simulink library "DCmotor_library"  (Simulink 7.4)
settings: Solver=ode45  StartTime=0.0  StopTime=10.0  RelTol=1e-3
libraries: simulink x4, rtsynclib x1
settings Model: Creator=ae  LastModifiedBy=sw

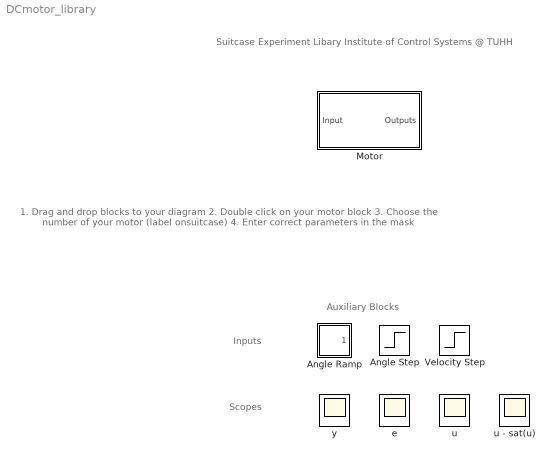
== system DCmotor_library ==
  note: Suitcase Experiment Libary
      | Institute of Control Systems @ TUHH
  note: 1. Drag and drop blocks to your diagram
      | 2. Double click on your motor block
      | 3. Choose the number of your motor (label onsuitcase)
      | 4. Enter correct parameters in the mask
  note: Auxiliary Blocks
  note: Inputs
  note: Scopes
  Angle Ramp : Subsystem  mask(Ramp){slope=1, start=1, X0=0, VectorParams1D=on, sampletime=0.01}
      mask prompts: slope "Simulink:masks:Slope_MP"; start "Simulink:masks:StartTime_MP"; X0 "Simulink:masks:InitialOutput_MP"; VectorParams1D "Simulink:masks:InterpretVectorParametersAs1D_MP"; sampletime "Sample time"
      mask help: Simulink:masks:Ramp_MD
      mask init:
      | blkName = gcb;
      | set_param([blkName '/Constant'], 'VectorParams1D',VectorParams1D);
      | set_param([blkName '/Constant1'], 'VectorParams1D',VectorParams1D);
      | set_param([blkName '/Step'], 'VectorParams1D',VectorParams1D);
      mask Display: plot([0:10],[1,1,1,1:8])
  Angle Step : Step  After=10  SampleTime=0.01
  Motor : Subsystem  InitFcn=|  StopFcn=|  mask{motoridinput=1, name_signal=Velocity, ts=10}
      InitFcn=|
      | id_tag = daq.getDevices().ID;
      | ni_obj = daq.createSession('ni');
      | ni_obj.addAnalogInputChannel(id_tag,'ai0','Voltage');
      | ni_obj.addAnalogInputChannel(id_tag,'ai1','Voltage');
      | ni_obj.addAnalogInputChannel(id_tag,'ai2','Voltage');
      | ni_obj.addAnalogInputChannel(id_tag,'ai3','Voltage');
      | ni_obj.addAnalogOutputChannel(id_tag, 'ao0', 'Voltage');
      StopFcn=|
      | ni_obj.outputSingleScan(2.5);          
      | clearvars ans id_tag jumps mvals ni_obj
      mask prompts: motoridinput "Motor Number"; name_signal "Output Variable"; ts "Sampling Time [ms]"
      mask help:
      | Select signal and corresponding units
      |
      |     Signal   |      SI     |      Motor
      | --------------------------------------------
      |    Velocity      [rad/s]         [rot/s]
      |    Angle          [rad]            [°]
      |    Current         [A]             [mA]
      |    Voltage         [V]             [V]
      mask init:
      | name_unit = 'SI'; %Motor, Raw
      | 
      | load motor.mat;
      | %global GLOB_motor
      | 
      | if ~exist('GLOB_motor')
      |     error('Please first load motor data from file motor.mat')
      | end
      | 
      | motor = GLOB_motor;
      | 
      | if strcmp(name_signal, 'Velocity')
      |     selector_signals = 1;
      | elseif strcmp(name_signal, 'Angle')
      |     selector_signals = 2;
      | elseif strcmp(name_signal, 'Current')
      |     selector_signals = 3;
      | elseif strcmp(name_signal, 'Voltage')
      |     selector_signals = 4;
      | else
      |     warning('using default: first signal')
      |     selector_signals = 1;
      | end
      | 
      | % setup DAQ object
      | % id_tag = daq.getDevices().ID;
      | % 
      | % ni_obj = daq.createSession('ni');
      | % 
      | % ni_obj.addAnalogInputChannel(id_tag,'ai0','Voltage');
      | % ni_obj.addAnalogInputChannel(id_tag,'ai1','Voltage');
      | % ni_obj.addAnalogInputChannel(id_tag,'ai2','Voltage');
      | % ni_obj.addAnalogInputChannel(id_tag,'ai3','Voltage');
      | % ni_obj.addAnalogOutputChannel(id_tag, 'ao0', 'Voltage');
      | 
      | % try
      | %    NIusb = visa('ni','USB::0x1234::125::A22-5::INSTR');
      | %    if ~strcmp(NIusb.ModelCode,'0x007D')
      | %        warning('Unknown NIDAQ model')
      | %    end
      | %    sn = NIusb.SerialNumber;
      | % catch
      | %    warning('USB device not detected automatically') 
      | %    sn = 0;
      | % end
      | % 
      | % 
      | % 
      | % if isnumeric(motoridinput)
      | %     if motoridinput == 31
      | %         if sn     
      | %             disp('Looking for known devices')
      | %             no = 1; 
      | %             while no < 31
      | %                 if strcmp(motor{no}.nidaq.serialnumber,sn)
      | %                     set_param(gcb,'motoridinput',num2str(no));
      | %                     break
      | %                 else
      | %                     no = no+1;
      | %                 end
      | %             end
      | %         else
      | %             warning('Motor could not be automatically detected - CALIBRATION for Motor 1 taken')
      | %             motorid = motor{1};
      | %         end
      | %         
      | %     elseif motoridinput == 0;
      | %   
      | %         motorid.calibration.velocity.offset = 0;
      | %         motorid.calibration.velocity.slope = 1;
      | %         motorid.calibration.angle.offset = 0;
      | %         motorid.calibration.angle.slope = 1;
      | %         motorid.calibration.current.offset = 0;
      | %         motorid.calibration.current.slope = 1;
      | %         motorid.calibration.voltage.offset = 0;
      | %         motorid.calibration.voltage.slope = 1;
      | %     elseif ((motoridinput == round(motoridinput)) & motoridinput <= 30)
      | %         if sn
      | %             if strcmp(motor{motoridinput}.nidaq.serialnumber,sn)
      | %                 motorid = motor{motoridinput};
      | %             else
      | %                 warning('Serial Number conflict: Wrong motor number given?')
      | %                 motorid = motor{motoridinput};
      | %             end
      | %         else
      | %             warning('Serial Number unknown: Calibration may be wrong')
      | %             motorid = motor{motoridinput}
      | %         end
      | %     else
      | %         error('Unknown motor ID')
      | %     end
      | % elseif isstruct(motoridinput)
      | %     disp('Using own motor ID structure')
      | % else
      | %     error('Wrong motor object - use motor number!')
      | % end
      | motorid = motor{motoridinput};
      | 
      | if strcmp(name_unit,'SI')
      |         motorid.calibration.velocity.unit = 1;
      |         motorid.calibration.angle.unit = 1;
      |         motorid.calibration.current.unit = 1;
      |         motorid.calibration.voltage.unit = 1;
      | elseif strcmp(name_unit,'Motor')
      |         motorid.calibration.velocity.unit = 2*pi;
      |         motorid.calibration.angle.unit = 180/pi;
      |         motorid.calibration.current.unit = 0.001;
      |         motorid.calibration.voltage.unit = 1;
      | elseif strcmp(name_unit,'Raw')
      |         motorid.calibration.velocity.unit = 1;
      |         motorid.calibration.angle.unit = 1;
      |         motorid.calibration.current.unit = 1;
      |         motorid.calibration.voltage.unit = 1;
      |         motorid.calibration.velocity.offset = 0;
      |         motorid.calibration.velocity.slope = 1;
      |         motorid.calibration.angle.offset = 0;
      |         motorid.calibration.angle.slope = 1;
      |         motorid.calibration.current.offset = 0;
      |         motorid.calibration.current.slope = 1;
      |         motorid.calibration.voltage.offset = 0;
      |         motorid.calibration.voltage.slope = 1;
      | else
      |     warning('Units not correct defined')
      | end
      | 
      | switch ts 
      |     % Sample Time
      |     case 1
      |         motorid.timing.sampletime = 10;
      |     case 2
      |         motorid.timing.sampletime = 20;
      |     case 3
      |         motorid.timing.sampletime = 30;
      |     case 4
      |         motorid.timing.sampletime = 50;
      |     case 5
      |         motorid.timing.sampletime = 75;
      |     case 6
      |         motorid.timing.sampletime = 100;
      |     case 7
      |         motorid.timing.sampletime = 150;
      |     otherwise
      |         error('unknown sampletime')
      | end
      | 
      | % Set the USB Port parameter
      | %tmp=daqhwinfo('nidaq');
      | 
      | %set_param([gcb,'/Analog Input'],'Device',['nidaq ' tmp.InstalledBoardIds{1} ' (USB-6008)']);
      | 
      | % Set the sampling rate
      | sr = motorid.timing.sampletime;
      | %set_param([gcb,'/motorzugriff'],'SampleRate',num2str(sr));
      | %   set_param([gcb,'/Analog Input'],'BlockSize','2');
      | 
      | 
      | % try 
      | %     % Initialize Adapter
      | %     hw = daqhwinfo;
      | %     adaptors = hw.InstalledAdaptors;
      | %     ni = daqhwinfo('nidaq');
      | %     id = ni.InstalledBoardIds;
      | %     name = ni.AdaptorName;
      | % 
      | %     % Find analog output
      | %     ao = analogoutput('nidaq',id{1});
      | %     set(ao,'SampleRate',ts);
      | %     ch = addchannel(ao,0);
      | % 
      | %     % Set corresponding motorid structure
      | %     motorid.signals.output = ao;
      | %     putsample(ao,2.5);
      | %     pause(3)
      | % catch
      | %     ao =[];
      | %     warning('No USB Board detected: Check connection')
      | % end
      mask StyleString: popup(1|2|3|4|5|6|7|8|9|10|11|12|13|14|15|16|17|18|19|20|21|22|23|24|25|26|27|28|29|30|31|32|33|34|35|36|37|38|39|40|41|42|43|44|45|46|47|48|49|50|51|52|53|54|55|56|57|58|59|60|61|62|unknown),popup(Velocity|Angle|Current|Voltage),popup(10|20|30|50|75|100|150)
      mask Display:
      | port_label('input', 1, 'Voltage')
      | port_label('output', 1, name_signal)
  Velocity Step : Step  After=47.75  SampleTime=0.01
  e : Scope
      settings: YMin=-0.5  YMax=11
  u : Scope
      settings: YMin=-0.5  YMax=11  SaveName=ScopeData2
  u - sat(u) : Scope
      settings: YMin=-0.5  YMax=11  SaveName=ScopeData3
  y : Scope
      settings: YMin=-0.5  YMax=11  SaveName=ScopeData4

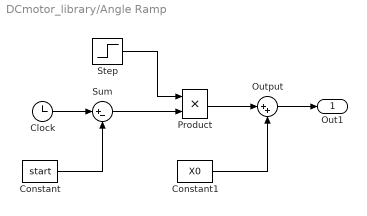
== system DCmotor_library/Angle Ramp ==
  Clock : Clock
      settings: DisableCoverage=on
  Constant : Constant  DisableCoverage=on  Value=start  OutDataTypeStr=Inherit: Inherit via back propagation
  Constant1 : Constant  DisableCoverage=on  Value=X0  OutDataTypeStr=Inherit: Inherit via back propagation
  Output : Sum  Inputs=|++  SaturateOnIntegerOverflow=on  InputSameDT=on  OutDataTypeStr=Inherit: Same as first input
  Product : Product  DisableCoverage=on  SaturateOnIntegerOverflow=on  InputSameDT=on  OutDataTypeStr=Inherit: Same as first input
  Step : Step  DisableCoverage=on  Time=start  After=slope  SampleTime=sampletime
  Sum : Sum  DisableCoverage=on  Inputs=|+-  SaturateOnIntegerOverflow=on  InputSameDT=on  OutDataTypeStr=Inherit: Same as first input
  Out1 : Outport
  wires:
  Clock/1 -> Sum/1
  Constant/1 -> Sum/2
  Sum/1 -> Product/2
  Output/1 -> Out1/1
  Constant1/1 -> Output/2
  Product/1 -> Output/1
  Step/1 -> Product/1

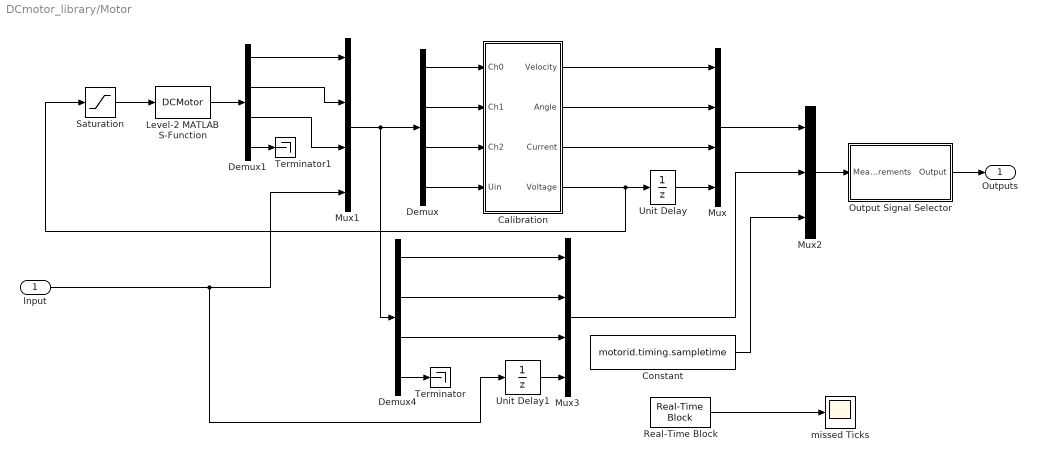
== system DCmotor_library/Motor ==
  Input : Inport
  Calibration : Subsystem
  Constant : Constant  Value=motorid.timing.sampletime
  Demux : Demux
  Demux1 : Demux
  Demux4 : Demux
  Level-2 MATLAB S-Function : M-S-Function  FunctionName=DCMotor  Parameters=ni_obj
  Mux : Mux
  Mux1 : Mux
  Mux2 : Mux  Inputs=3
  Mux3 : Mux
  Output Signal Selector : Subsystem  StopFcn=|
      | global GLOB_filename;        
      | %data.filename=GLOB_filename;
      | %data=save_data(data);
      mask Type: Output Signal Selector
      mask Description: Select the desired output.
      mask Display:
      | port_label('output',1, 'Output');
      | port_label('input' ,1 , 'Motor');
      | %port_label('input',1,['Task ' name_labproblem name_task name_subtask]);
  Real-Time Block : rtsynclib/Real-Time Block  sync_type=Fixed  sync_time=motorid.timing.sampletime*1e-3
  Saturation : Saturate  UpperLimit=5  LowerLimit=0
  Terminator : Terminator
  Terminator1 : Terminator
  Unit Delay : UnitDelay  SampleTime=-1
  Unit Delay1 : UnitDelay  SampleTime=-1
  missed Ticks : Scope
      settings: YMin=0  YMax=300
  Outputs : Outport
  wires:
  Demux4/4 -> Terminator/1
  Mux3/1 -> Mux2/2
  Unit Delay1/1 -> Mux3/4
  Demux4/3 -> Mux3/3
  Demux4/2 -> Mux3/2
  Demux4/1 -> Mux3/1
  Mux/1 -> Mux2/1
  Calibration/4(Voltage) -> Saturation/1, Unit Delay/1
  Calibration/3(Current) -> Mux/3
  Calibration/2(Angle) -> Mux/2
  Calibration/1(Velocity) -> Mux/1
  Mux1/1 -> Demux4/1, Demux/1
  Demux/1 -> Calibration/1(Ch0)
  Demux/2 -> Calibration/2(Ch1)
  Demux/3 -> Calibration/3(Ch2)
  Demux/4 -> Calibration/4(Uin)
  Demux1/1 -> Mux1/1
  Demux1/2 -> Mux1/2
  Demux1/3 -> Mux1/3
  Constant/1 -> Mux2/3
  Input/1 -> Unit Delay1/1, Mux1/4
  Unit Delay/1 -> Mux/4
  Real-Time Block/1 -> missed Ticks/1
  Mux2/1 -> Output Signal Selector/1(Measurements)
  Output Signal Selector/1(Output) -> Outputs/1
  Demux1/4 -> Terminator1/1
  Level-2 MATLAB S-Function/1 -> Demux1/1
  Saturation/1 -> Level-2 MATLAB S-Function/1

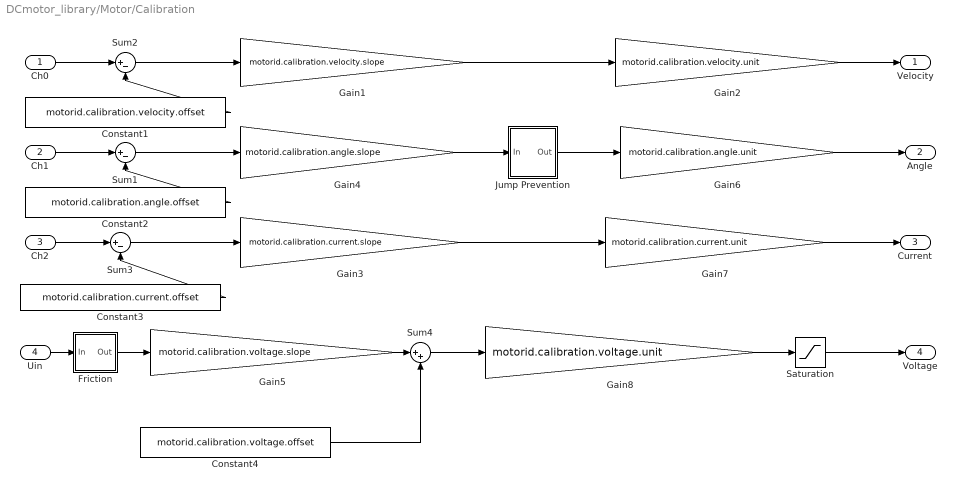
== system DCmotor_library/Motor/Calibration ==
  Ch0 : Inport
  Ch1 : Inport  Port=2
  Ch2 : Inport  Port=3
  Uin : Inport  Port=4
  Constant1 : Constant  Value=motorid.calibration.velocity.offset
  Constant2 : Constant  Value=motorid.calibration.angle.offset
  Constant3 : Constant  Value=motorid.calibration.current.offset
  Constant4 : Constant  Value=motorid.calibration.voltage.offset
  Friction : Subsystem
  Gain1 : Gain  Gain=motorid.calibration.velocity.slope
  Gain2 : Gain  Gain=motorid.calibration.velocity.unit
  Gain3 : Gain  Gain=motorid.calibration.current.slope
  Gain4 : Gain  Gain=motorid.calibration.angle.slope
  Gain5 : Gain  Gain=motorid.calibration.voltage.slope
  Gain6 : Gain  Gain=motorid.calibration.angle.unit
  Gain7 : Gain  Gain=motorid.calibration.current.unit
  Gain8 : Gain  Gain=motorid.calibration.voltage.unit
  Jump Prevention : Subsystem
  Saturation : Saturate  UpperLimit=5  LowerLimit=0
  Sum1 : Sum  Inputs=|+-
  Sum2 : Sum  Inputs=|+-
  Sum3 : Sum  Inputs=|+-
  Sum4 : Sum  Inputs=|++
  Velocity : Outport
  Angle : Outport  Port=2
  Current : Outport  Port=3
  Voltage : Outport  Port=4
  wires:
  Gain4/1 -> Jump Prevention/1(In)
  Gain8/1 -> Saturation/1
  Gain7/1 -> Current/1
  Gain6/1 -> Angle/1
  Gain2/1 -> Velocity/1
  Constant1/1 -> Sum2/2
  Constant2/1 -> Sum1/2
  Constant3/1 -> Sum3/2
  Constant4/1 -> Sum4/2
  Sum2/1 -> Gain1/1
  Ch0/1 -> Sum2/1
  Sum1/1 -> Gain4/1
  Ch1/1 -> Sum1/1
  Sum3/1 -> Gain3/1
  Ch2/1 -> Sum3/1
  Uin/1 -> Friction/1(In)
  Gain1/1 -> Gain2/1
  Gain3/1 -> Gain7/1
  Friction/1(Out) -> Gain5/1
  Sum4/1 -> Gain8/1
  Gain5/1 -> Sum4/1
  Saturation/1 -> Voltage/1
  Jump Prevention/1(Out) -> Gain6/1

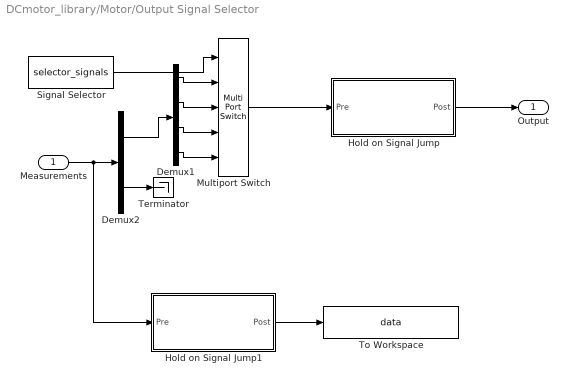
== system DCmotor_library/Motor/Output Signal Selector ==
  Measurements : Inport
  Demux1 : Demux
  Demux2 : Demux  Outputs=[4 -1]
  Hold on Signal Jump : Subsystem
  Hold on Signal Jump1 : Subsystem  AncestorBlock=DCmotor_library/Motor/Output Signal Selector/Hold on Signal Jump
  Multiport Switch : MultiPortSwitch  Inputs=4  zeroidx=off
  Signal Selector : Constant  Value=selector_signals
  Terminator : Terminator
  To Workspace : ToWorkspace  VariableName=data  SampleTime=-1  SaveFormat=Structure With Time
  Output : Outport
  wires:
  Multiport Switch/1 -> Hold on Signal Jump/1(Pre)
  Hold on Signal Jump/1(Post) -> Output/1
  Demux2/1 -> Demux1/1
  Measurements/1 -> Demux2/1, Hold on Signal Jump1/1(Pre)
  Demux1/1 -> Multiport Switch/2
  Demux1/2 -> Multiport Switch/3
  Demux1/3 -> Multiport Switch/4
  Demux1/4 -> Multiport Switch/5
  Signal Selector/1 -> Multiport Switch/1
  Demux2/2 -> Terminator/1
  Hold on Signal Jump1/1(Post) -> To Workspace/1

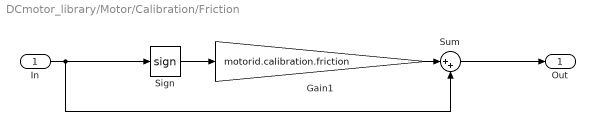
== system DCmotor_library/Motor/Calibration/Friction ==
  In : Inport
  Gain1 : Gain  DisableCoverage=on  Gain=motorid.calibration.friction  OutDataTypeStr=Inherit: Inherit via back propagation  SaturateOnIntegerOverflow=on
  Sign : Signum
  Sum : Sum  Inputs=|++  SaturateOnIntegerOverflow=on  InputSameDT=on  OutDataTypeStr=Inherit: Same as first input
  Out : Outport
  wires:
  Sum/1 -> Out/1
  Gain1/1 -> Sum/1
  In/1 -> Sign/1, Sum/2
  Sign/1 -> Gain1/1

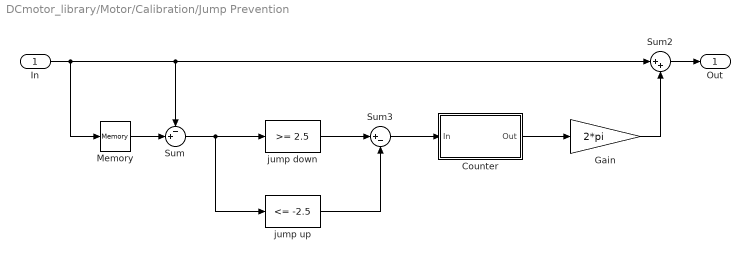
== system DCmotor_library/Motor/Calibration/Jump Prevention ==
  In : Inport
  Counter : Subsystem
  Gain : Gain  Gain=2*pi
  Memory : Memory
  Sum : Sum  Inputs=-+|
  Sum2 : Sum  Inputs=|++
  Sum3 : Sum  Inputs=|+-  OutDataTypeStr=double
  jump down : simulink/Logic and Bit Operations/Compare To Constant  relop=>=  const=2.5  LogicOutDataTypeMode=uint8  ZeroCross=off
  jump up : simulink/Logic and Bit Operations/Compare To Constant  relop=<=  const=-2.5  LogicOutDataTypeMode=uint8  ZeroCross=off
  Out : Outport
  wires:
  jump down/1 -> Sum3/1
  Sum2/1 -> Out/1
  Gain/1 -> Sum2/2
  jump up/1 -> Sum3/2
  Sum/1 -> jump up/1, jump down/1
  Memory/1 -> Sum/2
  In/1 -> Sum2/1, Sum/1, Memory/1
  Sum3/1 -> Counter/1(In)
  Counter/1(Out) -> Gain/1

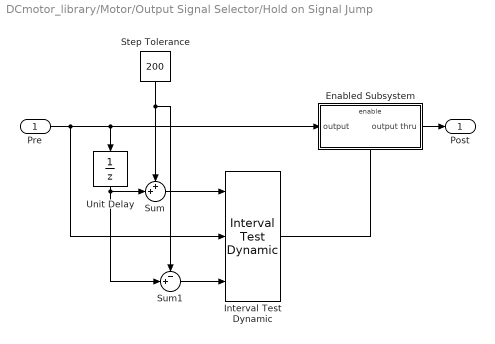
== system DCmotor_library/Motor/Output Signal Selector/Hold on Signal Jump ==
  Pre : Inport
  Enabled Subsystem : Subsystem  TreatAsAtomicUnit=on
  Interval Test Dynamic : simulink/Logic and Bit Operations/Interval Test Dynamic  IntervalClosedRight=on  IntervalClosedLeft=on  LogicOutDataTypeMode=boolean
  Step Tolerance : Constant  Value=200
  Sum : Sum  Inputs=++|
  Sum1 : Sum  Inputs=-+|
  Unit Delay : UnitDelay  SampleTime=-1
  Post : Outport
  wires:
  Enabled Subsystem/1(output thru) -> Post/1
  Pre/1 -> Enabled Subsystem/1(output), Unit Delay/1, Interval Test Dynamic/2
  Unit Delay/1 -> Sum/2, Sum1/2
  Sum/1 -> Interval Test Dynamic/1
  Sum1/1 -> Interval Test Dynamic/3
  Step Tolerance/1 -> Sum/1, Sum1/1
  Interval Test Dynamic/1 -> Enabled Subsystem/Enable

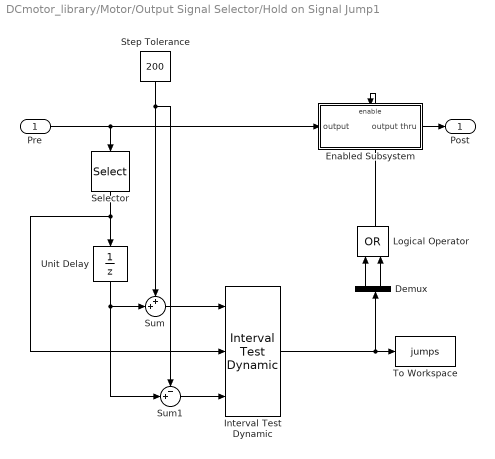
== system DCmotor_library/Motor/Output Signal Selector/Hold on Signal Jump1 ==
  Pre : Inport
  Demux : Demux  Outputs=2
  Enabled Subsystem : Subsystem  TreatAsAtomicUnit=on
  Interval Test Dynamic : simulink/Logic and Bit Operations/Interval Test Dynamic  IntervalClosedRight=on  IntervalClosedLeft=on  LogicOutDataTypeMode=boolean
  Logical Operator : Logic  Operator=OR  AllPortsSameDT=off  OutDataTypeStr=boolean
  Selector : Selector  InputPortWidth=9  IndexOptions=Index vector (dialog)  Indices=[1 2]  OutputSizes=1
  Step Tolerance : Constant  Value=200
  Sum : Sum  Inputs=++|
  Sum1 : Sum  Inputs=-+|
  To Workspace : ToWorkspace  VariableName=jumps  SampleTime=-1  SaveFormat=Structure
  Unit Delay : UnitDelay  SampleTime=-1
  Post : Outport
  wires:
  Interval Test Dynamic/1 -> To Workspace/1, Demux/1
  Step Tolerance/1 -> Sum1/1, Sum/1
  Sum1/1 -> Interval Test Dynamic/3
  Sum/1 -> Interval Test Dynamic/1
  Unit Delay/1 -> Sum1/2, Sum/2
  Pre/1 -> Enabled Subsystem/1(output), Selector/1
  Enabled Subsystem/1(output thru) -> Post/1
  Selector/1 -> Unit Delay/1, Interval Test Dynamic/2
  Demux/1 -> Logical Operator/1
  Demux/2 -> Logical Operator/2
  Logical Operator/1 -> Enabled Subsystem/Enable

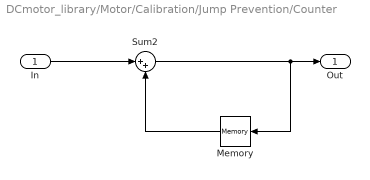
== system DCmotor_library/Motor/Calibration/Jump Prevention/Counter ==
  In : Inport
  Memory : Memory
  Sum2 : Sum  Inputs=|++
  Out : Outport
  wires:
  Sum2/1 -> Out/1, Memory/1
  In/1 -> Sum2/1
  Memory/1 -> Sum2/2

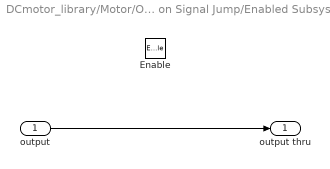
== system DCmotor_library/Motor/Output Signal Selector/Hold on Signal Jump/Enabled Subsystem ==
  output : Inport
  Enable : EnablePort  StatesWhenEnabling=reset  PropagateVarSize=During execution
  output thru : Outport
  wires:
  output/1 -> output thru/1

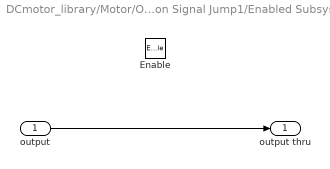
== system DCmotor_library/Motor/Output Signal Selector/Hold on Signal Jump1/Enabled Subsystem ==
  output : Inport
  Enable : EnablePort  StatesWhenEnabling=reset  PropagateVarSize=During execution
  output thru : Outport
  wires:
  output/1 -> output thru/1
